simulink model "enable_ex"  (R2020a)
settings: Solver=FixedStepAuto  StartTime=0.0  StopTime=10.0  FixedStep=0.001  MaxStep=0.001  RelTol=1e-3
libraries: simulink x1
settings Model: Creator=lenovo  LastModifiedBy=DELL
settings DataIOCC: ReturnWorkspaceOutputs=off
settings DebuggingCC: ArithmeticOperatorsInVariantConditions=warning
settings SFSimCC: SimUseLocalCustomCode=off  CustomCodeUndefinedFunction=UseInterfaceOnly
settings RTWCC: RTWUseLocalCustomCode=off

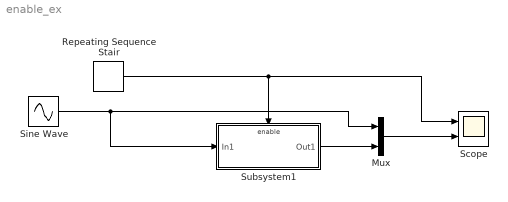
== system enable_ex ==
  Mux : Mux  Inputs=2
  Repeating Sequence Stair : simulink/Sources/Repeating Sequence Stair  OutValues=[-1 1].'  tsamp=1  OutMin=[]  OutMax=[]  OutDataTypeStr=double  OutputDataTypeScalingMode=double  OutDataType=fixdt(0,8)  ConRadixGroup=Best Precision: Vector-wise  OutScaling=2^-12
  Scope : Scope  NumInputPorts=2
  Sine Wave : Sin  SampleTime=0
  Subsystem1 : Subsystem
  wires:
  Repeating Sequence Stair/1 -> Subsystem1/Enable, Scope/1
  Sine Wave/1 -> Subsystem1/1(In1), Mux/1
  Subsystem1/1(Out1) -> Mux/2
  Mux/1 -> Scope/2

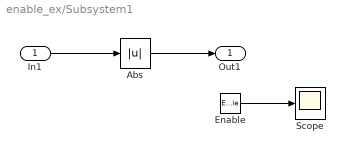
== system enable_ex/Subsystem1 ==
  In1 : Inport
  Enable : EnablePort  ShowOutputPort=on
  Abs : Abs
  Scope : Scope
  Out1 : Outport  VectorParamsAs1DForOutWhenUnconnected=off
  wires:
  Abs/1 -> Out1/1
  In1/1 -> Abs/1
  Enable/1 -> Scope/1
